simulink model "ES239A_HwAgCorrln"  (R2013b)
settings: Solver=FixedStepDiscrete  SolverMode=SingleTasking  StartTime=0.0  StopTime=1  FixedStep=0.002  RelTol=1e-3
values from neighbouring files (symbols this model uses):
  FLTINJ_HWAGCORRLN_HWAGIDPTSIG = DataDict.Constant    [ES239A_HwAgCorrln_DataDict.m]
  HwAgCorrlnHwAgAbsltDif = DataDict.Calibration    [ES239A_HwAgCorrln_DataDict.m]
  HwAgCorrlnHwAgMaxStall = DataDict.Calibration    [ES239A_HwAgCorrln_DataDict.m]
  HwAgCorrlnNtc0x092FailStep = DataDict.Calibration    [ES239A_HwAgCorrln_DataDict.m]
  HwAgCorrlnNtc0x092PassStep = DataDict.Calibration    [ES239A_HwAgCorrln_DataDict.m]
undefined symbols (not defined in the file or in its folder): NtcNr1, NtcSts1, sigbuilder_block
libraries: simulink x2, NxtrLim x2
(part 2 of 2)

== stateflow chart ES239A_HwAgCorrln/HwAgCorrln/HwAgCorrlnPer1/Correlation /Handwheel Angle Correlation Diagostic /SetNtcSts2/SetNtcSts/ISO Fault Debounce Design ==
  note: NTCSTS_PASSD           (0)
      | NTCSTS_FAILD             (1)
      | NTCSTS_PREPASSD   (2)
      | NTCSTS_PREFAILD     (3)
      |
      | SIGQLFR_NORES        (0)
      | SIGQLFR_PASSD         (1)
      | SIGQLFR_FAILD           (2)
  note: Pass Loop
  note: Fail Loop
  note: 
  (default) -> (junction 89)
  (junction 89) -> (junction 95) [order 1] : [NtcSts ==3]
  (junction 89) -> (junction 93) [order 2] : [NtcSts ==2]
  (junction 89) -> (junction 141) [order 3] : [NtcSts ==1]
      | { ErrAcc = 32767;
      | Qualifier =2;
      |  }
  (junction 89) -> (junction 141) [order 4] : [NtcSts ==0]
      | { ErrAcc = -32768;
      | Qualifier=1;
      | }
  (junction 95) -> (junction 103) [order 2]
  (junction 95) -> (junction 111) [order 1] : [ErrAcc <=0]
      | {ErrAcc = DebStep;}
  (junction 93) -> (junction 123) [order 2] : {
      | ErrAcc = ErrAcc - DebStep;
      | }
  (junction 93) -> (junction 123) [order 1] : [(ErrAcc - DebStep) <= -32768]
      | { ErrAcc = -32768;
      | Qualifier=1;
      | }
  (junction 103) -> (junction 111) [order 1] : [(ErrAcc + DebStep) <32767]
      | {ErrAcc = ErrAcc + DebStep;}
  (junction 103) -> (junction 111) [order 2] : {ErrAcc = 32767;
      | Qualifier =2;}
  (junction 123) -> (junction 141)
  (junction 111) -> (junction 141)
  (junction 141) -> (junction 159) [order 2] : {ErrAcc = 0;
      | Qualifier =0;
      | }
  (junction 141) -> (junction 159) [order 1] : [SvcClr ==0]
  data: NtcSts input Enum: NtcSts1; Qualifier output uint8; DebStep input uint16; ErrAcc local single; SvcClr input

== matlab function ES239A_HwAgCorrln/HwAgCorrln/HwAgCorrlnPer1/Correlation /Determine Number of Signals Valid ==
  data: HwAgAAvl input boolean; HwAgBAvl input boolean; NumberSignalsValid output uint8; LongTermCorrlnOk input uint8
function NumberSignalsValid = fcn(HwAgAAvl, HwAgBAvl, LongTermCorrlnOk)

aVarTruthTableCondition_1 = false;
aVarTruthTableCondition_2 = false;
aVarTruthTableCondition_3 = false;



aVarTruthTableCondition_1 = logical(HwAgAAvl);


aVarTruthTableCondition_2 = logical(HwAgBAvl);


aVarTruthTableCondition_3 = logical(LongTermCorrlnOk < 2);

if (aVarTruthTableCondition_1 && aVarTruthTableCondition_2 && aVarTruthTableCondition_3)
    aFcnTruthTableAction_1();
elseif (aVarTruthTableCondition_1 && aVarTruthTableCondition_2 && ~aVarTruthTableCondition_3)
    aFcnTruthTableAction_3();
elseif (~aVarTruthTableCondition_1 && ~aVarTruthTableCondition_2)
    aFcnTruthTableAction_3();
elseif (aVarTruthTableCondition_1 && ~aVarTruthTableCondition_2)
    aFcnTruthTableAction_2();
else % Default
    aFcnTruthTableAction_2();
end

function aFcnTruthTableAction_1()

% A and B are both valid

NumberSignalsValid = uint8(2);

function aFcnTruthTableAction_2()

% One Signal is Valid (A or B)

NumberSignalsValid = uint8(1);

function aFcnTruthTableAction_3()

% No Signals are Valid

NumberSignalsValid = uint8(0);

== stateflow chart ES239A_HwAgCorrln/HwAgCorrln/HwAgCorrlnPer1/Corrln Signal Availability/HwAgAAvlChk/CorrSigAvlChkRev1 ==
  note: SigAvl
      | False = 0
      | Pass = 1
  note: SigQlfr
      | 0 = No Result
      | 1 = Pass
      | 2 = Fail
  (default) -> (junction 2)
  (junction 2) -> (junction 4) [order 1] : [SigRollgCnt ==LstRollgCnt]
  (junction 4) -> (junction 7) [order 2] : {
      | StallCntOutp = LstStallCnt +1;
      | }
  (junction 2) -> (junction 3) [order 2]
  (junction 4) -> (junction 7) [order 1] : [LstStallCnt == 255]
      | {
      | StallCntOutp = 255;
      | }
  (junction 3) -> (junction 7) : {
      | StallCntOutp = 0;
      | }
  (junction 7) -> (junction 10)
  (junction 10) -> (junction 12) [order 1] : [StallCntOutp >=kMaxStallCnt]
  (junction 10) -> (junction 14) [order 2]
  (junction 12) -> (junction 17)
  (junction 14) -> (junction 17) [order 2]
  (junction 14) -> (junction 16) [order 1] : [SigQlfr<2]
  (junction 17) -> (junction 29) : {
      | SigAvl =0;
      | }
  (junction 16) -> (junction 29) : {
      | SigAvl = 1;
      | }
  data: SigRollgCnt input; SigQlfr input; kMaxStallCnt input; SigAvl output uint8; LstRollgCnt input uint8; LstStallCnt input uint8; StallCntOutp output uint8
